simulink model "contr1"  (Simulink 7.6)
settings: Solver=FixedStepDiscrete  StartTime=0.0  StopTime=2  FixedStep=1  RelTol=1e-3
libraries: simulink x3
settings Model: Creator=jordan  LastModifiedBy=jordan
settings DataIOCC: LimitDataPoints=off  SaveOutput=off  SignalLogging=off  DSMLogging=off  SaveTime=off
settings OptimizationCC: BlockReduction=off  ConditionallyExecuteInputs=off  InlineParams=on

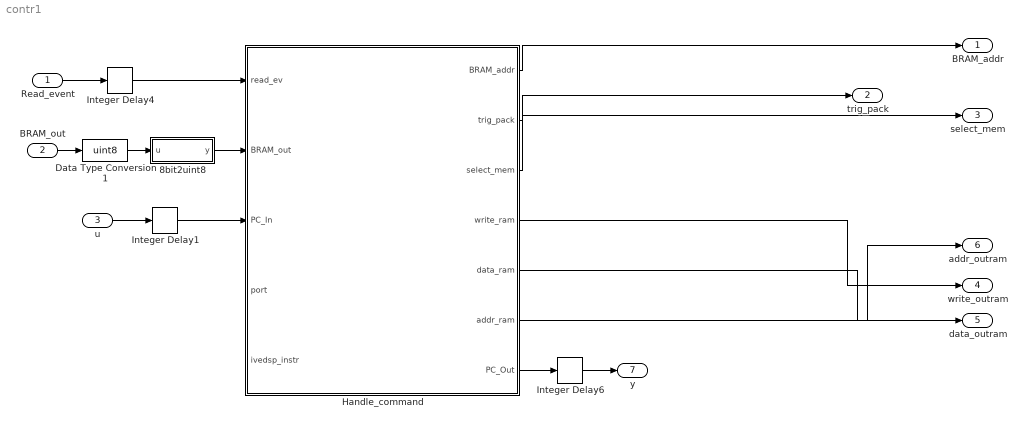
== system contr1 ==
  Read_event : Inport  OutDataTypeStr=boolean  PortDimensions=1
  BRAM_out : Inport  Port=2  OutDataTypeStr=boolean  PortDimensions=8
  u : Inport  Port=3
  8bit2uint8 : Stateflow chart  TreatAsAtomicUnit=on
  Data Type Conversion1 : DataTypeConversion  OutDataTypeStr=uint8
  Handle_command : Stateflow chart  TreatAsAtomicUnit=on
  Integer Delay1 : simulink/Discrete/Integer Delay  NumDelays=1  vinit=0.0  samptime=-1
  Integer Delay4 : simulink/Discrete/Integer Delay  NumDelays=1  vinit=0.0  samptime=-1
  Integer Delay6 : simulink/Discrete/Integer Delay  NumDelays=1  vinit=0.0  samptime=-1
  BRAM_addr : Outport
  trig_pack : Outport  Port=2
  select_mem : Outport  Port=3
  write_outram : Outport  Port=4
  data_outram : Outport  Port=5
  addr_outram : Outport  Port=6
  y : Outport  Port=7
  wires:
  Read_event/1 -> Integer Delay4/1
  BRAM_out/1 -> Data Type Conversion1/1
  Data Type Conversion1/1 -> 8bit2uint8/1(u)
  8bit2uint8/1(y) -> Handle_command/2(BRAM_out)
  Integer Delay4/1 -> Handle_command/1(read_ev)
  Handle_command/1(BRAM_addr) -> BRAM_addr/1
  Handle_command/2(trig_pack) -> trig_pack/1
  Handle_command/3(select_mem) -> select_mem/1
  Handle_command/4(write_ram) -> write_outram/1
  Handle_command/5(data_ram) -> data_outram/1
  Handle_command/6(addr_ram) -> addr_outram/1
  Handle_command/7(PC_Out) -> Integer Delay6/1
  u/1 -> Integer Delay1/1
  Integer Delay1/1 -> Handle_command/3(PC_In)
  Integer Delay6/1 -> y/1

== stateflow chart Handle_command ==
  settings: executeAtInitialization=1
  state Wait
  state Receive
  state Wait4
  state Wait2
  state Wait3
  state Wait8
  state Wait9
  (default) -> Receive
  (junction 11) -> Wait [order 2] : {ind++;
      | BRAM_addr=42+ind;
      | led=0;}
  Wait2 -> Receive : {BRAM_addr=0;
      | trig_pack=0;}
  Wait9 -> Wait8 : {addr_ram++;
      | data_ram=packet_out[addr_ram];}
  Wait -> Wait4
  Wait8 -> (junction 10) [order 1] : [addr_ram==15]
  (junction 11) -> (junction 13) [order 1] : [ind==16]
  (junction 12) -> Wait8 : {addr_ram=0;
      | write_ram=1;
      | data_ram=packet_out[addr_ram];}
  Wait8 -> Wait9 [order 2]
  (junction 13) -> (junction 10) [order 3]
  (junction 10) -> Wait2 : {write_ram=0;
      | select_mem=2;
      | trig_pack=1;}
  (junction 14) -> (junction 12) : {PC_Out_1[0]=packet[5];PC_Out_1[1]=packet[6];
      | PC_Out_2[0]=packet[7];PC_Out_2[1]=packet[8];
      | PC_Out_3[0]=packet[9];PC_Out_3[1]=packet[10];
      | PC_Out_4[0]=packet[11];PC_Out_4[1]=packet[12];
      | PC_Out_5[0]=packet[13];PC_Out_5[1]=packet[14];
      | PC_Out_6[0]=packet[15];PC_Out_6[1]=packet[16];}
  (junction 13) -> (junction 14) [order 1] : [packet[2]==LastCmd]{
      | LastCmd=LastCmd+1;
      | packet_out[1]=LastCmd;
      | packet_out[4]=PC_In_1[0];packet_out[5]=PC_In_1[1];
      | packet_out[6]=PC_In_1[2];packet_out[7]=PC_In_1[3];
      | packet_out[8]=PC_In_3[0];packet_out[9]=PC_In_3[1];
      | packet_out[10]=PC_In_4[0];packet_out[11]=PC_In_4[1];}
  Wait4 -> (junction 11) : {packet[ind]=BRAM_out;}
  (junction 13) -> Wait2 [order 2] : [packet[0]==6]{
      | select_mem=4;
      | trig_pack=1;}
      | /*ARP Request*/
  Receive -> Wait3 : [read_ev==1]{
      | BRAM_addr=14;}
  Wait3 -> Wait4 : {ind=0;}
  data: read_ev input boolean; BRAM_out input uint8; BRAM_addr output fixdt(0,11,0) =0; trig_pack output boolean; select_mem output fixdt(0,4,0) =0; ind local fixdt(0,5,0) =0; packet local uint8 size=17; LastCmd local uint8; packet_out local uint8 size=16; write_ram output boolean =0; data_ram output uint8; addr_ram output fixdt(0,14,0) =0; PC_In input uint8 size=4; PC_Out output uint8 size=4; port input fixdt(0,3,0); ivedsp_instr input boolean; ready local double

== matlab function 8bit2uint8 ==
  data: u input uint8 size=8; y output uint8
function y = fcn(u)
%#eml
y = uint8(bitor(bitor(bitor(bitor(bitor(bitor(bitor(u(8),bitshift(u(7),1)),bitshift(u(6),2)),bitshift(u(5),3)),bitshift(u(4),4)),bitshift(u(3),5)),bitshift(u(2),6)),bitshift(u(1),7)));
